simulink model "no_load_test_of_induction_motor"  (R2014b)
settings: Solver=ode23tb  StartTime=0.0  StopTime=5  MaxStep=1e-4  RelTol=1e-3
libraries: powerlib x13, powerlib_meascontrol x3
settings Model: Creator=Amr Saleh  LastModifiedBy=Amr Saleh

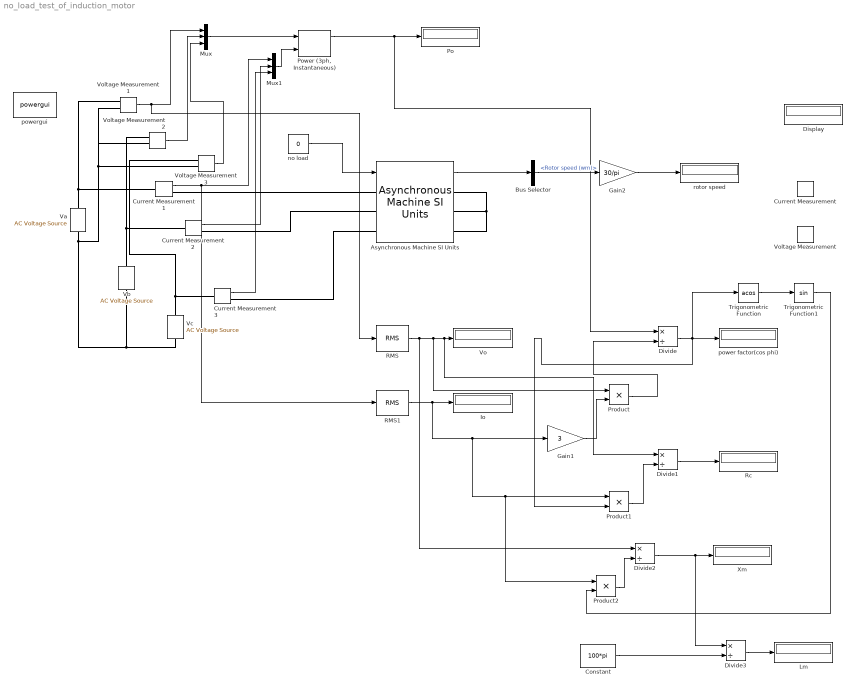
== system no_load_test_of_induction_motor ==
  Asynchronous Machine SI Units : powerlib/Machines/Asynchronous Machine SI Units  PresetModel=No  MechanicalLoad=Torque Tm  ShowDetailedParameters=on  RotorType=Wound  ReferenceFrame=Rotor  Units=SI  MeasurementBus=off  NominalParameters=[3.73e+04 460 50]  Stator=[0.09961 0.000867]  Rotor=[0.05837 0.000867]  Cage1=[ 0.022 0.226/377]  Cage2=[ 0.022 0.226/377]  Lm=0.03039  Mechanical=[0.4 0.02187 2]  PolePairs=2  InitialConditions=[1 0 0 0 0 0 0 0]  SimulateSaturation=off  Saturation=[14.03593122, 27.81365428, 53.79336849, 72.68890987, 97.98006896, 148.6815601, 215.7428561, 302.9841135, 420.4778367 ; 230, 322, 414, 460, 506, 552, 598, 644, 690]  LoadFlowParameters=1492000  TsPowergui=0  TsBlock=-1  IterativeModel=Trapezoidal non iterative  Pmec=0
  Bus Selector : BusSelector  OutputSignals=Mechanical.Rotor speed (wm)
  Constant : Constant  Value=100*pi
  Current Measurement{,1..3} (4 alike) : powerlib/Measurements/Current Measurement  PhasorSimulation=off  OutputType=Complex  PSBequivalent=0
  Display : Display
  Divide{,1..3} (4 alike) : Product  Inputs=*/
  Gain1 : Gain  Gain=3
  Gain2 : Gain  Gain=30/pi
  Io : Display
  Lm : Display
  Mux : Mux  Inputs=3
  Mux1 : Mux  Inputs=3
  Po : Display
  "Power (3ph, Instantaneous)" : powerlib_meascontrol/Measurements/Power (3ph, Instantaneous)
  Product : Product
  Product1 : Product
  Product2 : Product
  RMS : powerlib_meascontrol/Measurements/RMS  TrueRMS=off  Freq=50  RMSInit=0  Ts=0
  RMS1 : powerlib_meascontrol/Measurements/RMS  TrueRMS=off  Freq=50  RMSInit=0  Ts=0
  Rc : Display
  Trigonometric Function : Trigonometry  Operator=acos
  Trigonometric Function1 : Trigonometry
  Va : powerlib/Electrical Sources/AC Voltage Source  Amplitude=310  Phase=0  Frequency=50  SampleTime=0  Measurements=None
  Vb : powerlib/Electrical Sources/AC Voltage Source  Amplitude=310  Phase=-120  Frequency=50  SampleTime=0  Measurements=None
  Vc : powerlib/Electrical Sources/AC Voltage Source  Amplitude=310  Phase=120  Frequency=50  SampleTime=0  Measurements=None
  Vo : Display
  Voltage Measurement{,1..3} (4 alike) : powerlib/Measurements/Voltage Measurement  PhasorSimulation=off  OutputType=Complex  PSBequivalent=0
  Xm : Display
  no load : Constant  Value=0
  power factor(cos phi) : Display
  powergui : powerlib/powergui  Priority=1  SimulationMode=Continuous  SolverType=Tustin/Backward Euler (TBE)  SampleTime=50e-6  frequency=60  SPID=off  DisableSnubberDevices=off  DisableRonSwitches=off  DisableVfSwitches=off  SwTol=0  DisplayEquations=off  Interpol=off  methode=off  Ts=100  frequencyindice=50  Pbase=100e6  ErrMax=1e-4  Iterations=50  UnitsV=kV  UnitsW=MW  FunctionMessages=off  echomessages=off  HookPort=off  EnableUseOfTLC=off  x0status=blocks  RestoreLinks=warning  ResistiveCurrentMeasurement=off  Frange=[0:2:500]  Ylog=off  Xlog=on  ShowGrid=off  save=off  variable=ZData  structure=0  ZoomFFT=off  StartTime=0.0  cycles=1  DisplayStyle=1  fundamental=60  FreqAxis=off  MaxFrequency=1000  frequencyindicesteady=1  RmsSteady=1  display=off
  rotor speed : Display
  wires:
  no load/1 -> Asynchronous Machine SI Units/1
  Voltage Measurement1/1 -> RMS/1, Mux/1
  Voltage Measurement2/1 -> Mux/2
  Voltage Measurement3/1 -> Mux/3
  Mux/1 -> "Power (3ph, Instantaneous)"/1
  Current Measurement1/1 -> Mux1/1, RMS1/1
  Current Measurement2/1 -> Mux1/2
  Current Measurement3/1 -> Mux1/3
  Mux1/1 -> "Power (3ph, Instantaneous)"/2
  "Power (3ph, Instantaneous)"/1 -> Divide/1, Po/1
  RMS/1 -> Divide2/1, Product/1, Divide1/1, Vo/1
  RMS1/1 -> Product2/1, Product1/1, Gain1/1, Io/1
  Asynchronous Machine SI Units/1 -> Bus Selector/1
  Bus Selector/1 -> Gain2/1  "<Rotor speed (wm)>"
  Gain2/1 -> rotor speed/1
  Product/1 -> Divide/2
  Gain1/1 -> Product/2
  Divide/1 -> Trigonometric Function/1, Product1/2, power factor(cos phi)/1
  Product1/1 -> Divide1/2
  Divide1/1 -> Rc/1
  Trigonometric Function/1 -> Trigonometric Function1/1
  Trigonometric Function1/1 -> Product2/2
  Product2/1 -> Divide2/2
  Divide2/1 -> Divide3/1, Xm/1
  Constant/1 -> Divide3/2
  Divide3/1 -> Lm/1
  connections:
  Asynchronous Machine SI Units/RConn1 -- Asynchronous Machine SI Units/RConn2 -- Asynchronous Machine SI Units/RConn3
  Va/RConn1 -- Voltage Measurement1/LConn1 -- Current Measurement1/LConn1
  Current Measurement1/RConn1 -- Asynchronous Machine SI Units/LConn1
  Vb/RConn1 -- Current Measurement2/LConn1 -- Voltage Measurement2/LConn1
  Current Measurement2/RConn1 -- Asynchronous Machine SI Units/LConn2
  Vc/RConn1 -- Voltage Measurement3/LConn1 -- Current Measurement3/LConn1
  Current Measurement3/RConn1 -- Asynchronous Machine SI Units/LConn3
  Vc/LConn1 -- Voltage Measurement3/LConn2 -- Voltage Measurement2/LConn2 -- Voltage Measurement1/LConn2 -- Va/LConn1 -- Vb/LConn1
